simulink model "carriageway"  (R2021b)
settings: Solver=FixedStepAuto  StartTime=0.0  StopTime=10.0  RelTol=1e-3
settings Model: Creator=chioma  LastModifiedBy=chioma
settings ConfigComp: CovEnable=on  RecordCoverage=on  CovModelRefEnable=on

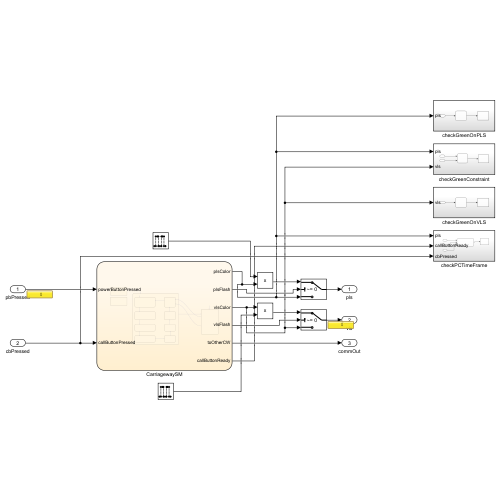
[thumbnail: Simulink's stored preview of the top-level diagram]
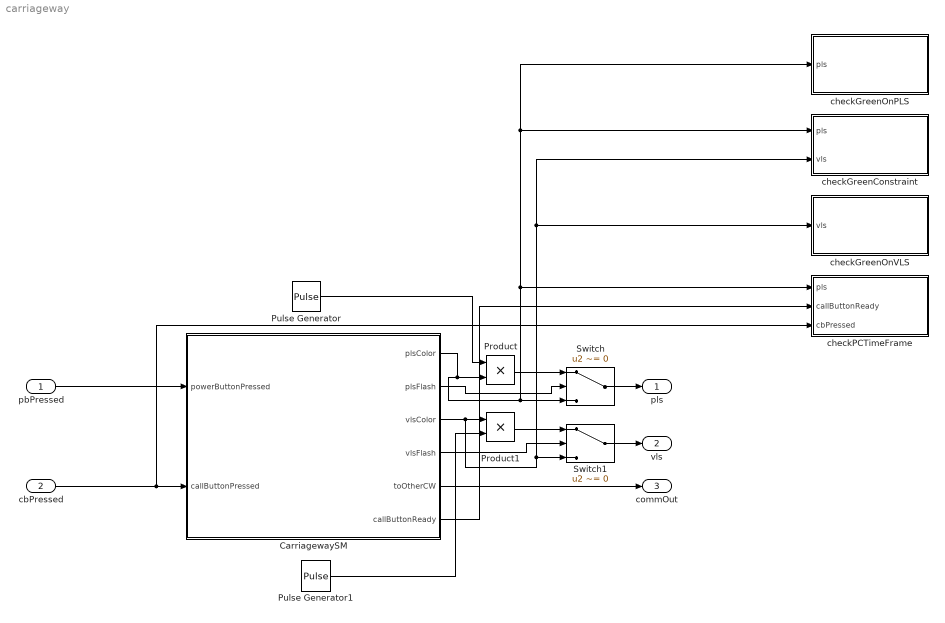
== system carriageway ==
  pbPressed : Inport
  cbPressed : Inport  Port=2
  CarriagewaySM : Stateflow chart  TreatAsAtomicUnit=on
  Product : Product
  Product1 : Product
  Pulse Generator : DiscretePulseGenerator
  Pulse Generator1 : DiscretePulseGenerator
  Switch : Switch  Criteria=u2 ~= 0  Threshold=1
  Switch1 : Switch  Criteria=u2 ~= 0  Threshold=1
  checkGreenConstraint : Subsystem
  checkGreenOnPLS : Subsystem
  checkGreenOnVLS : Subsystem
  checkPCTimeFrame : Subsystem
  pls : Outport
  vls : Outport  Port=2
  commOut : Outport  Port=3
  wires:
  Pulse Generator1/1 -> Product1/2
  Product1/1 -> Switch1/1
  Pulse Generator/1 -> Product/1
  Product/1 -> Switch/1
  CarriagewaySM/1(plsColor) -> Switch/3, checkGreenOnPLS/1(pls), checkGreenConstraint/1(pls), checkPCTimeFrame/1(pls), Product/2
  Switch/1 -> pls/1
  Switch1/1 -> vls/1
  CarriagewaySM/2(plsFlash) -> Switch/2
  CarriagewaySM/3(vlsColor) -> checkGreenConstraint/2(vls), checkGreenOnVLS/1(vls), Switch1/3, Product1/1
  CarriagewaySM/4(vlsFlash) -> Switch1/2
  pbPressed/1 -> CarriagewaySM/1(powerButtonPressed)
  cbPressed/1 -> checkPCTimeFrame/3(cbPressed), CarriagewaySM/2(callButtonPressed)
  CarriagewaySM/5(toOtherCW) -> commOut/1
  CarriagewaySM/6(callButtonReady) -> checkPCTimeFrame/2(callButtonReady)

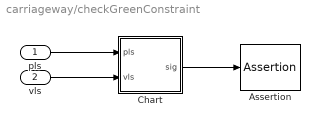
== system carriageway/checkGreenConstraint ==
  pls : Inport
  vls : Inport  Port=2
  Assertion : Assertion
  Chart : Stateflow chart  TreatAsAtomicUnit=on
  wires:
  Chart/1(sig) -> Assertion/1
  pls/1 -> Chart/1(pls)
  vls/1 -> Chart/2(vls)

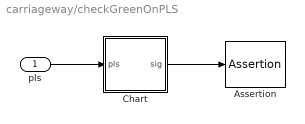
== system carriageway/checkGreenOnPLS ==
  pls : Inport
  Assertion : Assertion
  Chart : Stateflow chart  TreatAsAtomicUnit=on
  wires:
  Chart/1(sig) -> Assertion/1
  pls/1 -> Chart/1(pls)

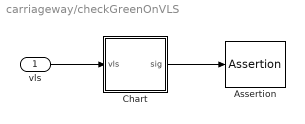
== system carriageway/checkGreenOnVLS ==
  vls : Inport
  Assertion : Assertion
  Chart : Stateflow chart  TreatAsAtomicUnit=on
  wires:
  Chart/1(sig) -> Assertion/1
  vls/1 -> Chart/1(vls)

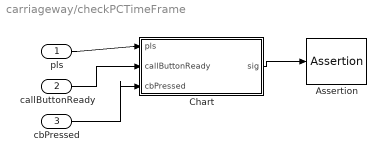
== system carriageway/checkPCTimeFrame ==
  pls : Inport
  callButtonReady : Inport  Port=2
  cbPressed : Inport  Port=3
  Assertion : Assertion
  Chart : Stateflow chart  TreatAsAtomicUnit=on
  wires:
  Chart/1(sig) -> Assertion/1
  pls/1 -> Chart/1(pls)
  callButtonReady/1 -> Chart/2(callButtonReady)
  cbPressed/1 -> Chart/3(cbPressed)

== stateflow chart carriageway/checkGreenOnPLS/Chart ==
  state handleAssertionEntry
    entry:
    sig = 1;
  state handleAssertionDuring
  state handleAssertionExit
    entry:
    sig = 0;
  (default) -> handleAssertionEntry
  handleAssertionEntry -> handleAssertionDuring : [pls == 2]
  handleAssertionDuring -> handleAssertionExit : before(x, sec)[pls ~= 2]
  data: sig output =1; pls input; x local =10

== stateflow chart carriageway/CarriagewaySM ==
  state VLS Color Code [group]
    note: Red => 1
        | Yellow => 2
        | Green => 3
  state on
    state vehiclesPassing
      entry:
      vlsColor = 3;
      vlsFlash = 0;
      plsColor = 1;
      plsFlash = 0;
      on after(10, sec):
      callButtonReady = 1;
    state vehiclesPassingReady
      entry:
      vlsColor = 2;
      vlsFlash = 0;
      plsColor = 1;
      plsFlash = 0;
    state vehiclesPassingSlowDown
      entry:
      vlsColor = 3;
      vlsFlash = 1;
      plsColor = 1;
      plsFlash = 0;
      callButtonReady = 0;
    state pedestriansCrossingDone
      entry:
      vlsColor = 1;
      vlsFlash = 0;
      plsColor = 1;
      plsFlash = 0;
    state vehiclesPassingAlmostDone
      entry:
      vlsColor = 2;
      vlsFlash = 0;
      plsColor = 1;
      plsFlash = 0;
      toOtherCW = 1;
    state pedestriansCrossingAlmostDone
      entry:
      vlsColor = 1;
      vlsFlash = 0;
      plsColor = 2;
      plsFlash = 1;
    state vehiclesPassingDone
      entry:
      vlsColor = 1;
      vlsFlash = 0;
      plsColor = 1;
      plsFlash = 0;
      toOtherCW = 0;
    state pedestriansCrossing
      entry:
      vlsColor = 1;
      vlsFlash = 0;
      plsColor = 2;
      plsFlash = 0;
    (default) -> vehiclesPassing
    vehiclesPassingReady -> vehiclesPassing : after(3, sec)
    vehiclesPassing -> vehiclesPassingSlowDown : [callButtonPressed && callButtonReady == 1]
    pedestriansCrossingDone -> vehiclesPassingReady : after(3, sec)
    vehiclesPassingSlowDown -> vehiclesPassingAlmostDone : after(5, sec)
    pedestriansCrossingAlmostDone -> pedestriansCrossingDone : after(5, sec)
    vehiclesPassingAlmostDone -> vehiclesPassingDone : after(3, sec)
    pedestriansCrossing -> pedestriansCrossingAlmostDone : after(10, sec)
    vehiclesPassingDone -> pedestriansCrossing : after(3, sec)
  state PLS Color Code [group]
    note: Red => 1
        | Green => 2
  state off
    entry:
    vlsColor = 0;
    vlsFlash = 0;
    plsColor = 0;
    plsFlash = 0;
    during:
    timer = timer + 1;
  (default) -> on [order 2]
  off -> vehiclesPassingReady [order 2] : [powerButtonPressed == 1 && timer > 3]
  off -> vehiclesPassingReady [order 1] : after(10, sec)[powerButtonPressed == 1 && timer <= 3]
  (default) -> off [order 1] : [powerButtonPressed == 0]
  on -> off : [powerButtonPressed == 0]
  data: powerButtonPressed input; plsColor output =0; plsFlash output; vlsColor output =0; vlsFlash output; timer local =0; callButtonPressed input boolean; toOtherCW output =0; callButtonReady output =0

== stateflow chart carriageway/checkGreenOnVLS/Chart ==
  state handleAssertionEntry
    entry:
    sig = 1;
  state handleAssertionDuring
  state handleAssertionExit
    entry:
    sig = 0;
  (default) -> handleAssertionEntry
  handleAssertionEntry -> handleAssertionDuring : [vls == 3]
  handleAssertionDuring -> handleAssertionExit : before(y, sec)[vls ~= 3]
  data: sig output =1; vls input; y local =10

== stateflow chart carriageway/checkPCTimeFrame/Chart ==
  state handleAssertionEntry
    entry:
    sig = 1;
    timer = 0;
  state handleAssertionDuring
    during:
    timer = timer + 1;
  state handleAssertionExit
    entry:
    sig = 0;
  (default) -> handleAssertionEntry
  (junction 17) -> handleAssertionEntry [order 2] : [timer <= z]
  handleAssertionEntry -> handleAssertionDuring : [cbPressed]
  handleAssertionDuring -> (junction 17) : [pls == 2]
  (junction 17) -> handleAssertionExit [order 1] : [timer > z]
  data: sig output =1; pls input; z local =12; timer local; callButtonReady input; cbPressed input

== stateflow chart carriageway/checkGreenConstraint/Chart ==
  state handleAssertionEntry
    entry:
    sig = 1;
  state handleAssertionDuring
    sig = 0;
  (default) -> handleAssertionEntry
  handleAssertionEntry -> handleAssertionDuring : [vls == 3 && pls == 2]
  data: sig output =1; pls input; vls input
